simulink model "tank_model"  (R2019b)
settings: Solver=FixedStepAuto  StartTime=0.0  StopTime=15  FixedStep=0.1  RelTol=1e-3
values from neighbouring files (symbols this model uses):
  den = 900    [defx.m]    (also in initial_pa_mixtank.m)
  V = 1    [defx.m]    (also in initial_pa_mixtank.m)
  x1 = 0.4    [defx.m]    (also in initial_pa_mixtank.m)
  x2 = 0.75    [defx.m]    (also in initial_pa_mixtank.m)
settings Model: Creator=luong  LastModifiedBy=luong

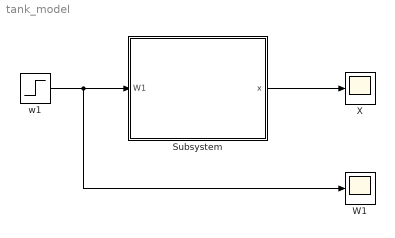
== system tank_model ==
  Subsystem : Subsystem
  W1 : Scope
  X : Scope
  w1 : Step  Time=5  Before=500  After=400  SampleTime=0
  wires:
  w1/1 -> W1/1, Subsystem/1(W1)
  Subsystem/1(x) -> X/1

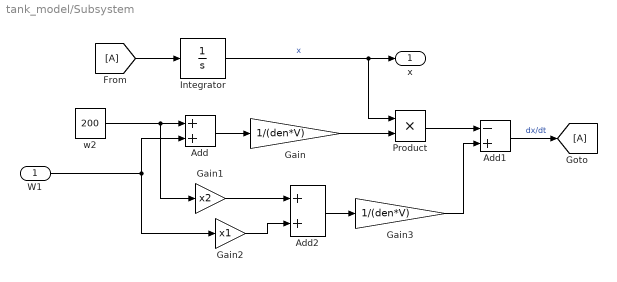
== system tank_model/Subsystem ==
  W1 : Inport
  Add : Sum
  Add1 : Sum  Inputs=-+
  Add2 : Sum
  Gain : Gain  Gain=1/(den*V)
  Gain1 : Gain  Gain=x2
  Gain2 : Gain  Gain=x1
  Gain3 : Gain  Gain=1/(den*V)
  Integrator : Integrator  InitialCondition=0.5
  Product : Product
  w2 : Constant  Value=200
  x : Outport
  wires:
  w2/1 -> Gain1/1, Add/1
  Add/1 -> Gain/1
  Integrator/1 -> x/1, Product/1  "x"
  W1/1 -> Gain2/1, Add/2
  Add2/1 -> Gain3/1
  Gain2/1 -> Add2/2
  Gain/1 -> Product/2
  Product/1 -> Add1/1
  Gain1/1 -> Add2/1
  Gain3/1 -> Add1/2
  Add1/1 -> [A]  "dx/dt"
  [A] -> Integrator/1
